simulink model "CaccavaleVillani"  (R2014b)
settings: Solver=ode1  SolverMode=SingleTasking  StartTime=0.0  StopTime=3  RelTol=1e-3
values from neighbouring files (symbols this model uses):
  alpha = 1.5    [CaViInit.m]    (also in CaccavaleVillani.m = 2)
  d1 = 1000    [CaViInit.m]    (also in CaccavaleVillani.m = 100)
  delta1 = 80    [CaViInit.m]    (also in CaccavaleVillani.m = 100)
  deltao = 10    [CaViInit.m]    (also in CaccavaleVillani.m = 2000)
  Do = 1500    [CaViInit.m]    (also in CaccavaleVillani.m = 2000)
  g = [0;0;-9.81]    [CaViInit.m]    (also in CaccavaleVillani.m)
  j0 = 0.2    [CaViInit.m]    (also in CaccavaleVillani.m = 1)
  j1 = 2    [CaViInit.m]    (also in CaccavaleVillani.m = 1)
  j1d = 1.00*j1    (= 2)    [CaViInit.m]    (also in CaccavaleVillani.m = 1)
  j2 = 2    [CaViInit.m]    (also in CaccavaleVillani.m = 1)
  j2d = 1.00*j2    (= 2)    [CaViInit.m]    (also in CaccavaleVillani.m = 1)
  j3 = 2    [CaViInit.m]    (also in CaccavaleVillani.m = 1)
  j3d = 1.00*j3    (= 2)    [CaViInit.m]    (also in CaccavaleVillani.m = 1)
  j4 = 2    [CaViInit.m]    (also in CaccavaleVillani.m = 1)
  j4d = 1.00*j4    (= 2)    [CaViInit.m]    (also in CaccavaleVillani.m = 1)
  k1 = 400    [CaViInit.m]    (also in CaccavaleVillani.m = 10000)
  K_o = 700    [CaViInit.m]    (also in CaccavaleVillani.m = 10000)
  kappa1 = 2    [CaViInit.m]    (also in CaccavaleVillani.m = 250)
  kappa_o = 5    [CaViInit.m]    (also in CaccavaleVillani.m = 10000)
  kpr = 150    [CaViInit.m]    (also in CaccavaleVillani.m = 10000)
  kpt = 50    [CaViInit.m]    (also in CaccavaleVillani.m = 50000)
  kvr = 14    [CaViInit.m]
  kvt = 192    [CaViInit.m]
  m0 = 1.4    [CaViInit.m]    (also in CaccavaleVillani.m = 10)
  m1 = 2    [CaViInit.m]    (also in CaccavaleVillani.m = 10)
  m1d = 1.00*m1    (= 2)    [CaViInit.m]    (also in CaccavaleVillani.m = 10)
  m2 = 2    [CaViInit.m]    (also in CaccavaleVillani.m = 10)
  m2d = 1.00*m2    (= 2)    [CaViInit.m]    (also in CaccavaleVillani.m = 10)
  m3 = 2    [CaViInit.m]    (also in CaccavaleVillani.m = 10)
  m3d = 1.00*m3    (= 2)    [CaViInit.m]    (also in CaccavaleVillani.m = 10)
  m4 = 2    [CaViInit.m]    (also in CaccavaleVillani.m = 10)
  m4d = 1.00*m4    (= 2)    [CaViInit.m]    (also in CaccavaleVillani.m = 10)
  r = 0.4*[1; 0; 0 ... (first row only)    [CaViInit.m]    (also in CaccavaleVillani.m = [1; 0; 0)
libraries: aerolibutil x26, aerolibtransform2 x3, dspinverses x3, simulink x2
(part 2 of 2)

== system CaccavaleVillani/Positional Control/Subsystem/Subsystem1 ==
  x_r2 : Inport
  x2 : Inport  Port=2
  Add2 : Sum  Inputs=+-
  Demux4 : Demux
  Demux5 : Demux  Outputs=7
  Demux6 : Demux  Outputs=7
  Mux5 : Mux
  Mux6 : Mux  Inputs=3
  Mux7 : Mux
  Mux8 : Mux  Inputs=3
  Mux9 : Mux
  Prod1 : Product  Multiplication=Matrix(*)
  Quaternion Division2 : aerolibutil/Quaternion Division
  k1; 2kappa1*eta2 : MATLAB Function  TreatAsAtomicUnit=on
  hk2 : Outport
  wires:
  Demux5/6 -> Mux7/3
  Demux6/1 -> Mux8/1
  x_r2/1 -> Demux5/1
  Demux6/3 -> Mux8/3
  Demux6/2 -> Mux8/2
  Demux6/5 -> Mux9/2
  Demux6/4 -> Mux9/1
  Demux6/7 -> Mux9/4
  Demux6/6 -> Mux9/3
  Mux6/1 -> Add2/1
  x2/1 -> Demux6/1
  Mux7/1 -> Quaternion Division2/1
  Mux8/1 -> Add2/2
  Add2/1 -> Mux5/1
  Mux9/1 -> Quaternion Division2/2
  k1; 2kappa1*eta2/1(K) -> Prod1/1
  Demux4/1 -> k1; 2kappa1*eta2/1(eta2)
  Mux5/1 -> Prod1/2
  Quaternion Division2/1 -> Demux4/1
  Prod1/1 -> hk2/1
  Demux4/4 -> Mux5/4
  Demux4/3 -> Mux5/3
  Demux4/2 -> Mux5/2
  Demux5/1 -> Mux6/1
  Demux5/2 -> Mux6/2
  Demux5/3 -> Mux6/3
  Demux5/4 -> Mux7/1
  Demux5/7 -> Mux7/4
  Demux5/5 -> Mux7/2

== system CaccavaleVillani/Positional Control/Subsystem/Subsystem2 ==
  x_r3 : Inport
  x3 : Inport  Port=2
  Add3 : Sum  Inputs=+-
  Demux7 : Demux
  Demux8 : Demux  Outputs=7
  Demux9 : Demux  Outputs=7
  Mux10 : Mux
  Mux11 : Mux  Inputs=3
  Mux12 : Mux
  Mux13 : Mux  Inputs=3
  Mux14 : Mux
  Prod2 : Product  Multiplication=Matrix(*)
  Quaternion Division3 : aerolibutil/Quaternion Division
  k1; 2kappa1*eta3 : MATLAB Function  TreatAsAtomicUnit=on
  hk3 : Outport
  wires:
  Demux7/1 -> k1; 2kappa1*eta3/1(eta3)
  Prod2/1 -> hk3/1
  Demux8/1 -> Mux11/1
  Demux7/3 -> Mux10/3
  Demux7/2 -> Mux10/2
  Quaternion Division3/1 -> Demux7/1
  Mux10/1 -> Prod2/2
  Demux7/4 -> Mux10/4
  Demux8/7 -> Mux12/4
  Demux9/2 -> Mux13/2
  Demux9/1 -> Mux13/1
  Demux8/2 -> Mux11/2
  Demux8/3 -> Mux11/3
  Demux8/4 -> Mux12/1
  x_r3/1 -> Demux8/1
  Demux8/5 -> Mux12/2
  Demux8/6 -> Mux12/3
  Demux9/5 -> Mux14/2
  Demux9/7 -> Mux14/4
  Mux11/1 -> Add3/1
  k1; 2kappa1*eta3/1(K) -> Prod2/1
  x3/1 -> Demux9/1
  Add3/1 -> Mux10/1
  Mux13/1 -> Add3/2
  Mux12/1 -> Quaternion Division3/1
  Mux14/1 -> Quaternion Division3/2
  Demux9/4 -> Mux14/1
  Demux9/3 -> Mux13/3
  Demux9/6 -> Mux14/3

== system CaccavaleVillani/Positional Control/Subsystem/Subsystem3 ==
  x_r4 : Inport
  x4 : Inport  Port=2
  Add4 : Sum  Inputs=+-
  Demux10 : Demux
  Demux11 : Demux  Outputs=7
  Demux12 : Demux  Outputs=7
  Mux15 : Mux
  Mux16 : Mux  Inputs=3
  Mux17 : Mux
  Mux18 : Mux  Inputs=3
  Mux19 : Mux
  Prod3 : Product  Multiplication=Matrix(*)
  Quaternion Division4 : aerolibutil/Quaternion Division
  k1; 2kappa1*eta4 : MATLAB Function  TreatAsAtomicUnit=on
  hk4 : Outport
  wires:
  k1; 2kappa1*eta4/1(K) -> Prod3/1
  Demux10/1 -> k1; 2kappa1*eta4/1(eta4)
  Mux15/1 -> Prod3/2
  Quaternion Division4/1 -> Demux10/1
  Prod3/1 -> hk4/1
  Demux10/4 -> Mux15/4
  Demux10/3 -> Mux15/3
  Demux10/2 -> Mux15/2
  Demux11/1 -> Mux16/1
  Demux11/2 -> Mux16/2
  Demux11/3 -> Mux16/3
  Demux11/4 -> Mux17/1
  Demux11/5 -> Mux17/2
  Demux11/6 -> Mux17/3
  Demux11/7 -> Mux17/4
  x_r4/1 -> Demux11/1
  Demux12/1 -> Mux18/1
  Demux12/2 -> Mux18/2
  Demux12/3 -> Mux18/3
  Demux12/4 -> Mux19/1
  Demux12/5 -> Mux19/2
  Demux12/6 -> Mux19/3
  Demux12/7 -> Mux19/4
  x4/1 -> Demux12/1
  Mux16/1 -> Add4/1
  Mux18/1 -> Add4/2
  Mux17/1 -> Quaternion Division4/1
  Mux19/1 -> Quaternion Division4/2
  Add4/1 -> Mux15/1

== matlab function CaccavaleVillani/Reference Trajectory/MATLAB Function1 ==
  data: eta_o input; K output; K_o parameter; kappa_o parameter
function K = stiffness(eta_o,K_o,kappa_o)
K = blkdiag(K_o*eye(3),2*eta_o*kappa_o*eye(3));

== matlab function CaccavaleVillani/Reference Trajectory/Grasp Matrix ==
  data: r parameter; G output; x input size=28
function G = GraspMatrix(r,x)
%x_o = [eye(3) zeros(3,4) eye(3) zeros(3,4) eye(3) zeros(3,4) eye(3) zeros(3,4)] * x;
G = [eye(3) zeros(3) eye(3) zeros(3) eye(3) zeros(3) eye(3) zeros(3);
    skew_sm(quatrot(x(4:7),r(1:3))) eye(3) skew_sm(quatrot(x(4:7),r(4:6))) eye(3) skew_sm(quatrot(x(4:7),r(7:9))) eye(3) skew_sm(quatrot(x(4:7),r(10:12))) eye(3)];

== matlab function CaccavaleVillani/Reference Trajectory/Coriolis Force ==
  data: dx_do input; hcoriolis output; j0 parameter; m0 parameter
function hcoriolis = CoriolisForce(dx_do,j0,m0)
hcoriolis = [m0*skew_sm(dx_do(4:6))*dx_do(1:3);
        j0*skew_sm(dx_do(4:6))*dx_do(4:6)];

== matlab function CaccavaleVillani/Impedance control/Reduced Constraint Matrix ==
  data: r parameter; Ared output; x input
function Ared = ReducedConstraintMAtrix(r,x)
%x_o = [eye(3) zeros(3,4) eye(3) zeros(3,4) eye(3) zeros(3,4) eye(3) zeros(3,4)] * x;
Ared = [-eye(3) skew_sm(quatrot(x(4:7),r(4:6)-r(1:3))) eye(3) zeros(3,15);
        zeros(3) -eye(3) zeros(3) eye(3) zeros(3,12);
        -eye(3) skew_sm(quatrot(x(4:7),r(7:9)-r(1:3))) zeros(3,6) eye(3) zeros(3,9);
        zeros(3) -eye(3) zeros(3,9) eye(3) zeros(3,6);
        -eye(3) skew_sm(quatrot(x(4:7),r(10:12)-r(1:3))) zeros(3,12) eye(3) zeros(3);
        zeros(3) -eye(3) zeros(3,15) eye(3)];
% Ared = [-eye(3) skew_sm(quatrot(x(4:7),x(8:10)-x(1:3))) eye(3) zeros(3,15);
%         zeros(3) -eye(3) zeros(3) eye(3) zeros(3,12);
%         -eye(3) skew_sm(quatrot(x(4:7),x(15:17)-x(1:3))) zeros(3,6) eye(3) zeros(3,9);
%         zeros(3) -eye(3) zeros(3,9) eye(3) zeros(3,6);
%         -eye(3) skew_sm(quatrot(x(4:7),x(22:24)-x(1:3))) zeros(3,12) eye(3) zeros(3);
%         zeros(3) -eye(3) zeros(3,15) eye(3)];

== matlab function CaccavaleVillani/Interaction dynamics1/MATLAB Function ==
  data: r parameter; A output; x input
function A = ConstraintMatrix(r,x)
A = [-eye(3) skew_sm(quatrot(x(4:7),r(1:3))) eye(3) zeros(3,21);
        zeros(3) -eye(3) zeros(3) eye(3) zeros(3,18);
        -eye(3) skew_sm(quatrot(x(4:7),r(4:6))) zeros(3,6) eye(3) zeros(3,15);
        zeros(3) -eye(3) zeros(3,9) eye(3) zeros(3,12);
        -eye(3) skew_sm(quatrot(x(4:7),r(7:9))) zeros(3,12) eye(3) zeros(3,9);
        zeros(3) -eye(3) zeros(3,15) eye(3) zeros(3,6);
        -eye(3) skew_sm(quatrot(x(4:7),r(10:12))) zeros(3,18) eye(3) zeros(3);
        zeros(3) -eye(3) zeros(3,21) eye(3)];

== matlab function CaccavaleVillani/Interaction dynamics1/Centripetal Force ==
  data: dx input; b output; r parameter; x input
function b = centripetalforce(dx,r,x)
b = [skew_sm(dx(4:6))*skew_sm(dx(4:6))*quatrot(x(4:7),r(1:3));
     zeros(3,1);
     skew_sm(dx(4:6))*skew_sm(dx(4:6))*quatrot(x(4:7),r(4:6));
     zeros(3,1);
     skew_sm(dx(4:6))*skew_sm(dx(4:6))*quatrot(x(4:7),r(7:9));
     zeros(3,1);
     skew_sm(dx(4:6))*skew_sm(dx(4:6))*quatrot(x(4:7),r(10:12));
     zeros(3,1)];

== matlab function CaccavaleVillani/Interaction dynamics1/Coriolis Force ==
  data: dx input; hcoriolis output; j0 parameter; m0 parameter
function hcoriolis = CoriolisForce(dx,j0,m0)
hcoriolis = [m0*skew_sm(dx(4:6))*dx(1:3);
        j0*skew_sm(dx(4:6))*dx(4:6)];

== matlab function CaccavaleVillani/Impedance control/Manipulator 2/k1; 2kappa1*eta2 ==
  data: eta1 input; K output; k1 parameter; kappa1 parameter
function K = stiffness(eta1,k1,kappa1)
K = blkdiag(k1*eye(3),2*eta1*kappa1*eye(3));

== matlab function CaccavaleVillani/Impedance control/Manipulator 3/k1; 2kappa1*eta3 ==
  data: eta1 input; K output; k1 parameter; kappa1 parameter
function K = stiffness(eta1,k1,kappa1)
K = blkdiag(k1*eye(3),2*eta1*kappa1*eye(3));

== matlab function CaccavaleVillani/Impedance control/Manipulator 4/k1; 2kappa1*eta4 ==
  data: eta1 input; K output; k1 parameter; kappa1 parameter
function K = stiffness(eta1,k1,kappa1)
K = blkdiag(k1*eye(3),2*eta1*kappa1*eye(3));

== matlab function CaccavaleVillani/Reference Trajectory/VIrtual Object Dynamics/Coriolis Force ==
  data: dx_do input; hcoriolis output; j0 parameter; m0 parameter
function hcoriolis = CoriolisForce(dx_do,j0,m0)
hcoriolis = [m0*skew_sm(dx_do(4:6))*dx_do(1:3);
        j0*skew_sm(dx_do(4:6))*dx_do(4:6)];

== matlab function CaccavaleVillani/Positional Control/Subsystem/Subsystem/k1; 2kappa1*eta1 ==
  data: eta1 input; kpt parameter; kpr parameter; K output
function K = stiffness(eta1,kpt,kpr)
K = blkdiag(kpt*eye(3),2*eta1*kpr*eye(3));

== matlab function CaccavaleVillani/Positional Control/Subsystem/Subsystem1/k1; 2kappa1*eta2 ==
  data: eta2 input; kpt parameter; K output; kpr parameter
function K = stiffness(eta2,kpt,kpr)
K = blkdiag(kpt*eye(3),2*eta2*kpr*eye(3));

== matlab function CaccavaleVillani/Positional Control/Subsystem/Subsystem2/k1; 2kappa1*eta3 ==
  data: eta3 input; kpt parameter; K output; kpr parameter
function K = stiffness(eta3,kpt,kpr)
K = blkdiag(kpt*eye(3),2*eta3*kpr*eye(3));

== matlab function CaccavaleVillani/Positional Control/Subsystem/Subsystem3/k1; 2kappa1*eta4 ==
  data: eta4 input; kpt parameter; K output; kpr parameter
function K = stiffness(eta4,kpt,kpr)
K = blkdiag(kpt*eye(3),2*eta4*kpr*eye(3));

== matlab function CaccavaleVillani/Kinematic Coordination/Grasp Matrix ==
  data: r parameter; G output; x input
function G = GraspMatrix(r,x)
%x_o = [eye(3) zeros(3,4) eye(3) zeros(3,4) eye(3) zeros(3,4) eye(3) zeros(3,4)] * x;
G = [eye(3) zeros(3) eye(3) zeros(3) eye(3) zeros(3) eye(3) zeros(3);
    skew_sm(quatrot(x(4:7),r(1:3))) eye(3) skew_sm(quatrot(x(4:7),r(4:6))) eye(3) skew_sm(quatrot(x(4:7),r(7:9))) eye(3) skew_sm(quatrot(x(4:7),r(10:12))) eye(3)];

== matlab function CaccavaleVillani/Kinematic Coordination/Manipulator Position//Orientation in World Frame ==
  data: p_do input size=3; q_do input size=4; x_d output; r parameter
function x_d = manipulatorpose(p_do,q_do,r)

x_d = [p_do + quatrot(q_do,r(1:3));
        q_do;
        p_do + quatrot(q_do,r(4:6));
        q_do;
        p_do + quatrot(q_do,r(7:9));
        q_do;
        p_do + quatrot(q_do,r(10:12));
        q_do];

== matlab function CaccavaleVillani/Kinematic Coordination/Centripetal Force ==
  data: dx_do input; b output; x input; r parameter
function b = centripetalforce(dx_do,x,r)
%x_o = [eye(3) zeros(3,4) eye(3) zeros(3,4) eye(3) zeros(3,4) eye(3) zeros(3,4)] * x;
b = [skew_sm(dx_do(4:6))*skew_sm(dx_do(4:6))*quatrot(x(4:7),r(1:3));
     zeros(3,1);
     skew_sm(dx_do(4:6))*skew_sm(dx_do(4:6))*quatrot(x(4:7),r(4:6));
     zeros(3,1);
     skew_sm(dx_do(4:6))*skew_sm(dx_do(4:6))*quatrot(x(4:7),r(7:9));
     zeros(3,1);
     skew_sm(dx_do(4:6))*skew_sm(dx_do(4:6))*quatrot(x(4:7),r(10:12));
     zeros(3,1)];

== matlab function CaccavaleVillani/Impedance control/Manipulator 1/k1; 2kappa1*eta1 ==
  data: eta1 input; K output; k1 parameter; kappa1 parameter
function K = stiffness(eta1,k1,kappa1)
K = blkdiag(k1*eye(3),2*eta1*kappa1*eye(3));

== matlab function CaccavaleVillani/Manipulator dynamics/Reduced Constraint Matrix ==
  data: r parameter; Ared output; x input
function Ared = ReducedConstraintMAtrix(r,x)
%x_o = [eye(3) zeros(3,4) eye(3) zeros(3,4) eye(3) zeros(3,4) eye(3) zeros(3,4)] * x;
Ared = [-eye(3) skew_sm(quatrot(x(4:7),r(4:6)-r(1:3))) eye(3) zeros(3,15);
        zeros(3) -eye(3) zeros(3) eye(3) zeros(3,12);
        -eye(3) skew_sm(quatrot(x(4:7),r(7:9)-r(1:3))) zeros(3,6) eye(3) zeros(3,9);
        zeros(3) -eye(3) zeros(3,9) eye(3) zeros(3,6);
        -eye(3) skew_sm(quatrot(x(4:7),r(10:12)-r(1:3))) zeros(3,12) eye(3) zeros(3);
        zeros(3) -eye(3) zeros(3,15) eye(3)];
% Ared = [-eye(3) skew_sm(quatrot(x(4:7),x(8:10)-x(1:3))) eye(3) zeros(3,15);
%         zeros(3) -eye(3) zeros(3) eye(3) zeros(3,12);
%         -eye(3) skew_sm(quatrot(x(4:7),x(15:17)-x(1:3))) zeros(3,6) eye(3) zeros(3,9);
%         zeros(3) -eye(3) zeros(3,9) eye(3) zeros(3,6);
%         -eye(3) skew_sm(quatrot(x(4:7),x(22:24)-x(1:3))) zeros(3,12) eye(3) zeros(3);
%         zeros(3) -eye(3) zeros(3,15) eye(3)];

== matlab function CaccavaleVillani/Manipulator dynamics/Centripal Force ==
  data: r parameter; x input; bred output; dx input
function bred = ReducedCentripetalvector(r,x,dx)
bred = [skew_sm(dx(4:6))*skew_sm(dx(4:6))*quatrot(x(4:7),(r(4:6)-r(1:3)));
        zeros(3,1);
        skew_sm(dx(4:6))*skew_sm(dx(4:6))*quatrot(x(4:7),(r(7:9)-r(1:3)));
        zeros(3,1);
        skew_sm(dx(4:6))*skew_sm(dx(4:6))*quatrot(x(4:7),(r(10:12)-r(1:3)));
        zeros(3,1)];
%     bred = [skew_sm(dx(4:6))*skew_sm(dx(4:6))*quatrot(x(4:7),(x(8:10)-x(1:3)));
%         zeros(3,1);
%         skew_sm(dx(4:6))*skew_sm(dx(4:6))*quatrot(x(4:7),(x(15:17)-x(1:3)));
%         zeros(3,1);
%         skew_sm(dx(4:6))*skew_sm(dx(4:6))*quatrot(x(4:7),(x(22:24)-x(1:3)));
%         zeros(3,1)];

== matlab function CaccavaleVillani/Interaction dynamics/Apparent Inertia ==
  data: G input; Mapp output; M input; m0 parameter; j0 parameter
function Mapp = ApparentInertia(G,M,m0,j0)
Mapp = blkdiag(m0*eye(3),j0*eye(3)) + G*M*G';

== matlab function CaccavaleVillani/Interaction dynamics/Grasp Matrix ==
  data: r parameter; G output; x input
function G = GraspMatrix(r,x)
G = [eye(3) zeros(3) eye(3) zeros(3) eye(3) zeros(3) eye(3) zeros(3);
    skew_sm(quatrot(x(4:7),r(1:3))) eye(3) skew_sm(quatrot(x(4:7),r(4:6))) eye(3) skew_sm(quatrot(x(4:7),r(7:9))) eye(3) skew_sm(quatrot(x(4:7),r(10:12))) eye(3)];

== matlab function CaccavaleVillani/Interaction dynamics/Coriolis Force ==
  data: dx input; hcoriolis output; j0 parameter; m0 parameter
function hcoriolis = CoriolisForce(dx,j0,m0)
hcoriolis = [m0*skew_sm(dx(4:6))*dx(1:3);
        j0*skew_sm(dx(4:6))*dx(4:6)];

== matlab function CaccavaleVillani/Interaction dynamics/Centripetal Force ==
  data: dx input; b output; r parameter; x input
function b = centripetalforce(dx,r,x)
b = [skew_sm(dx(4:6))*skew_sm(dx(4:6))*quatrot(x(4:7),r(1:3));
     zeros(3,1);
     skew_sm(dx(4:6))*skew_sm(dx(4:6))*quatrot(x(4:7),r(4:6));
     zeros(3,1);
     skew_sm(dx(4:6))*skew_sm(dx(4:6))*quatrot(x(4:7),r(7:9));
     zeros(3,1);
     skew_sm(dx(4:6))*skew_sm(dx(4:6))*quatrot(x(4:7),r(10:12));
     zeros(3,1)];

== matlab function CaccavaleVillani/Manipulator motion/Grasp Matrix ==
  data: r parameter; G output; x input
function G = GraspMatrix(r,x)
G = [eye(3) zeros(3) eye(3) zeros(3) eye(3) zeros(3) eye(3) zeros(3);
    skew_sm(quatrot(x(4:7),r(1:3))) eye(3) skew_sm(quatrot(x(4:7),r(4:6))) eye(3) skew_sm(quatrot(x(4:7),r(7:9))) eye(3) skew_sm(quatrot(x(4:7),r(10:12))) eye(3)];

== matlab function CaccavaleVillani/Manipulator motion/Manipualtor pose in world frame ==
  data: p_o input; q_o input size=4; x output; r parameter
function x = manipulatorpose(p_o,q_o,r)

x = [p_o + quatrot(q_o,r(1:3));
        q_o;
        p_o + quatrot(q_o,r(4:6));
        q_o;
        p_o + quatrot(q_o,r(7:9));
        q_o;
        p_o + quatrot(q_o,r(10:12));
        q_o ];

== matlab function CaccavaleVillani/Allocator/MATLAB Function1 ==
  data: r parameter; bred output; dx input; x input
function bred = ReducedCentripetalvector(r,dx,x)
% bred = [skew_sm(dx(4:6))*skew_sm(dx(4:6))*quatrot(x(4:7),r(4:6)-r(1:3));
%     zeros(3,1);
%     skew_sm(dx(4:6))*skew_sm(dx(4:6))*quatrot(x(4:7),r(7:9)-r(1:3));
%     zeros(3,1);
%     skew_sm(dx(4:6))*skew_sm(dx(4:6))*quatrot(x(4:7),r(10:12)-r(1:3));
%     zeros(3,1)];
    bred = [skew_sm(dx(4:6))*skew_sm(dx(4:6))*quatrot(x(4:7),(x(8:10)-x(1:3)));
        zeros(3,1);
        skew_sm(dx(4:6))*skew_sm(dx(4:6))*quatrot(x(4:7),(x(15:17)-x(1:3)));
        zeros(3,1);
        skew_sm(dx(4:6))*skew_sm(dx(4:6))*quatrot(x(4:7),(x(22:24)-x(1:3)));
        zeros(3,1)];

== matlab function CaccavaleVillani/Allocator/MATLAB Function ==
  data: r parameter; Ared output; x input
function Ared = ReducedConstraintMAtrix(r,x)
% Ared = [-eye(3) skew_sm(quatrot(x(4:7),r(4:6)-r(1:3))) eye(3) zeros(3,15);
%         zeros(3) -eye(3) zeros(3) eye(3) zeros(3,12);
%         -eye(3) skew_sm(quatrot(x(4:7),r(7:9)-r(1:3))) zeros(3,6) eye(3) zeros(3,9);
%         zeros(3) -eye(3) zeros(3,9) eye(3) zeros(3,6);
%         -eye(3) skew_sm(quatrot(x(4:7),r(10:12)-r(1:3))) zeros(3,12) eye(3) zeros(3);
%         zeros(3) -eye(3) zeros(3,15) eye(3)];
Ared = [-eye(3) skew_sm(quatrot(x(4:7),x(8:10)-x(1:3))) eye(3) zeros(3,15);
        zeros(3) -eye(3) zeros(3) eye(3) zeros(3,12);
        -eye(3) skew_sm(quatrot(x(4:7),x(15:17)-x(1:3))) zeros(3,6) eye(3) zeros(3,9);
        zeros(3) -eye(3) zeros(3,9) eye(3) zeros(3,6);
        -eye(3) skew_sm(quatrot(x(4:7),x(22:24)-x(1:3))) zeros(3,12) eye(3) zeros(3);
        zeros(3) -eye(3) zeros(3,15) eye(3)];

== matlab function CaccavaleVillani/Manipulator dynamics/World to Object Frame ==
  data: hw input; x input; h_int output
function h_int = inertial2objectFrame(hw,x)

h_int = [quatrot(quatconj(x(4:7)')',hw(1:3));
         hw(4:6);%quatrot(quatconj(x(4:7)')',hw(4:6));
         quatrot(quatconj(x(4:7)')',hw(7:9));
         hw(10:12);%quatrot(quatconj(x(4:7)')',hw(10:12));
         quatrot(quatconj(x(4:7)')',hw(13:15));
         hw(16:18);%quatrot(quatconj(x(4:7)')',hw(16:18));
         quatrot(quatconj(x(4:7)')',hw(19:21));
         hw(22:24)];%quatrot(quatconj(x(4:7)')',hw(22:24));];
